simulink model "GyroModel"  (R2018b)
settings: Solver=ode3  StartTime=0.0  StopTime=180  FixedStep=1/1000  RelTol=1e-3
undefined symbols (not defined in the file): w, wn, z, zeta
libraries: simulink x1
settings Model: Creator=rachellecheung  LastModifiedBy=rachellecheung

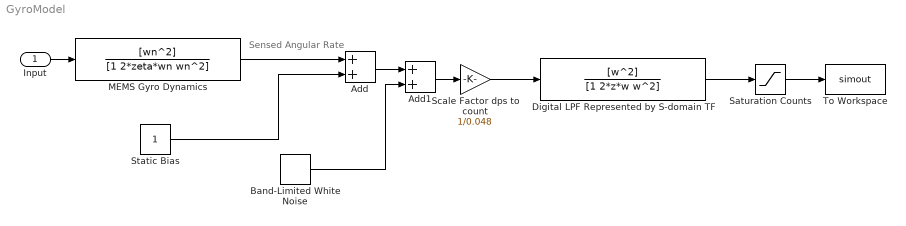
== system GyroModel ==
  note: Sensed Angular Rate
  Input : Inport
  Add : Sum
  Add1 : Sum
  Band-Limited White Noise : simulink/Sources/Band-Limited White Noise  Cov=[0.018^2]  Ts=1/1000  seed=[23341]
  Digital LPF Represented by S-domain TF : TransferFcn  Numerator=[w^2]  Denominator=[1 2*z*w w^2]
  MEMS Gyro Dynamics : TransferFcn  Numerator=[wn^2]  Denominator=[1 2*zeta*wn wn^2]
  Saturation Counts : Saturate  UpperLimit=2^15  LowerLimit=-2^15
  Scale Factor dps to count : Gain  Gain=1/0.048
  Static Bias : Constant
  To Workspace : ToWorkspace  VariableName=simout  SampleTime=-1
  wires:
  MEMS Gyro Dynamics/1 -> Add/1
  Add/1 -> Add1/1
  Static Bias/1 -> Add/2
  Band-Limited White Noise/1 -> Add1/2
  Add1/1 -> Scale Factor dps to count/1
  Saturation Counts/1 -> To Workspace/1
  Scale Factor dps to count/1 -> Digital LPF Represented by S-domain TF/1
  Input/1 -> MEMS Gyro Dynamics/1
  Digital LPF Represented by S-domain TF/1 -> Saturation Counts/1
